simulink model "test_yL_epsL"  (R2018a)
settings: Solver=ode23  StartTime=0.0  StopTime=tend  FixedStep=0.01  RelTol=1e-3  EnableMultiTasking=on
values from neighbouring files (symbols this model uses):
  delta = @(u) 0.0015*(u-t0)*(u>t0) - 0.0035*(u-t1)*(u>t1)    [test_yL_epsL_.m]
undefined symbols (not defined in the file or in its folder): pin
libraries: SLlib_lka_thesis x6, simulink_extras x1, simulink x1
settings Model: Creator=Georg  LastModifiedBy=georgnestlinger
settings DataIOCC: LimitDataPoints=on  SaveFormat=Array  SignalLoggingSaveFormat=ModelDataLogs
settings OptimizationCC: DefaultParameterBehavior=Inlined  ExpressionDepthLimit=2147483647  LifeSpan=inf
settings DebuggingCC: UnderspecifiedInitializationDetection=Classic  MergeDetectMultiDrivingBlocksExec=none  StateNameClashWarn=warning  SFUnexpectedBacktrackingDiag=warning  SFNoUnconditionalDefaultTransitionDiag=warning  SFExecutionAtInitializationDiag=none
settings HardwareCC: ProdBitPerPointer=32  ProdBitPerSizeT=32  ProdBitPerPtrDiffT=32  ProdLargestAtomicFloat=None  ProdIntDivRoundTo=Undefined  ProdEndianess=Unspecified  ProdWordSize=32  ProdHWDeviceType=32-bit Generic
settings ModelReferenceCC: PropagateSignalLabelsOutOfModel=off
settings CodeAppCC: StateflowObjectComments=on
settings GRTTargetCC: TargetLangStandard=C89/C90 (ANSI)  GeneratePreprocessorConditionals=Disable all  CombineOutputUpdateFcns=off  GRTInterface=on
settings ConfigComp: CovMetricSettings=dw  CovHtmlReporting=on  CovSaveCumulativeToWorkspaceVar=on  CovSaveSingleToWorkspaceVar=on  CovExternalEMLEnable=off

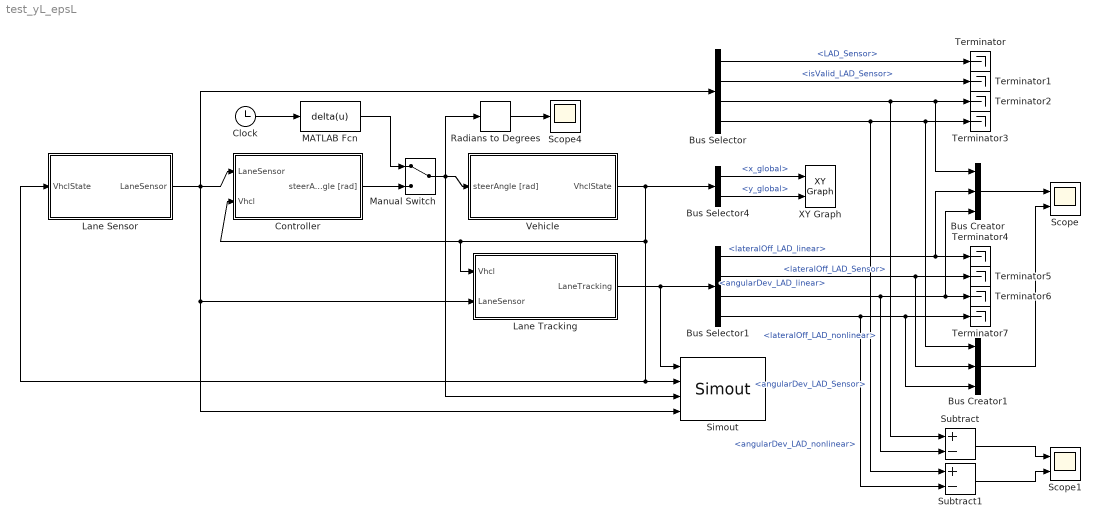
== system test_yL_epsL ==
  Bus Creator : BusCreator  Inputs=3
  Bus Creator1 : BusCreator  Inputs=3
  Bus Selector : BusSelector  OutputSignals=LAD_Sensor,isValid_LAD_Sensor,lateralOff_LAD_Sensor,angularDev_LAD_Sensor
  Bus Selector1 : BusSelector  OutputSignals=lateralOff_LAD_linear,angularDev_LAD_linear,lateralOff_LAD_nonlinear,angularDev_LAD_nonlinear
  Bus Selector4 : BusSelector  OutputSignals=x_global,y_global
  Clock : Clock
  Controller : Subsystem
  Lane Sensor : Subsystem
  Lane Tracking : Subsystem
  MATLAB Fcn : MATLABFcn  MATLABFcn=delta(u)
  Manual Switch : ManualSwitch
  Radians to Degrees : simulink_extras/Transformations/Radians to Degrees
  Scope : Scope  NumInputPorts=2
  Scope1 : Scope  NumInputPorts=2
  Scope4 : Scope
  Simout : SLlib_lka_thesis/Misc/Simout
  Subtract : Sum  Inputs=+-
  Subtract1 : Sum  Inputs=+-
  Terminator{,1..7} (8 alike) : Terminator
  Vehicle : Subsystem
  XY Graph : simulink/Sinks/XY Graph  xmin=-50  xmax=700  ymin=-10  ymax=600  st=-1
  wires:
  MATLAB Fcn/1 -> Manual Switch/1
  Clock/1 -> MATLAB Fcn/1
  Radians to Degrees/1 -> Scope4/1
  Manual Switch/1 -> Vehicle/1(steerAngle [rad]), Radians to Degrees/1, Simout/3
  Controller/1(steerAngle [rad]) -> Manual Switch/2
  Vehicle/1(VhclState) -> Bus Selector4/1, Lane Tracking/1(Vhcl), Controller/2(Vhcl), Simout/2, Lane Sensor/1(VhclState)
  Lane Sensor/1(LaneSensor) -> Controller/1(LaneSensor), Bus Selector/1, Lane Tracking/2(LaneSensor), Simout/4
  Bus Selector4/1 -> XY Graph/1  "<x_global>"
  Bus Selector4/2 -> XY Graph/2  "<y_global>"
  Bus Creator1/1 -> Scope/2
  Bus Creator/1 -> Scope/1
  Lane Tracking/1(LaneTracking) -> Bus Selector1/1, Simout/1
  Bus Selector/1 -> Terminator/1  "<LAD_Sensor>"
  Bus Selector/2 -> Terminator1/1  "<isValid_LAD_Sensor>"
  Bus Selector/3 -> Terminator2/1, Bus Creator/1, Subtract/1  "<lateralOff_LAD_Sensor>"
  Bus Selector/4 -> Terminator3/1, Bus Creator1/1, Subtract1/1  "<angularDev_LAD_Sensor>"
  Bus Selector1/1 -> Terminator4/1, Bus Creator/2  "<lateralOff_LAD_linear>"
  Bus Selector1/2 -> Terminator5/1, Bus Creator1/2  "<angularDev_LAD_linear>"
  Bus Selector1/3 -> Terminator6/1, Bus Creator/3, Subtract/2  "<lateralOff_LAD_nonlinear>"
  Bus Selector1/4 -> Terminator7/1, Bus Creator1/3, Subtract1/2  "<angularDev_LAD_nonlinear>"
  Subtract1/1 -> Scope1/2
  Subtract/1 -> Scope1/1

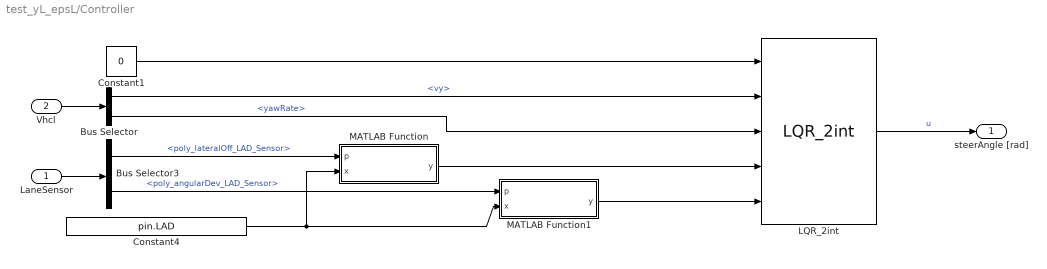
== system test_yL_epsL/Controller ==
  LaneSensor : Inport
  Vhcl : Inport  Port=2
  Bus Selector : BusSelector  OutputSignals=vy,yawRate
  Bus Selector3 : BusSelector  OutputSignals=poly_lateralOff_LAD_Sensor,poly_angularDev_LAD_Sensor
  Constant1 : Constant  Value=0
  Constant4 : Constant  Value=pin.LAD
  LQR_2int : SLlib_lka_thesis/LKA-Controller/LQR_2int
  MATLAB Function : MATLAB Function  TreatAsAtomicUnit=on
  MATLAB Function1 : MATLAB Function  TreatAsAtomicUnit=on
  steerAngle [rad] : Outport
  wires:
  Constant1/1 -> LQR_2int/1
  MATLAB Function/1(y) -> LQR_2int/4
  MATLAB Function1/1(y) -> LQR_2int/5
  Constant4/1 -> MATLAB Function1/2(x), MATLAB Function/2(x)
  LaneSensor/1 -> Bus Selector3/1
  LQR_2int/1 -> steerAngle [rad]/1  "u"
  Bus Selector3/1 -> MATLAB Function/1(p)  "<poly_lateralOff_LAD_Sensor>"
  Bus Selector3/2 -> MATLAB Function1/1(p)  "<poly_angularDev_LAD_Sensor>"
  Vhcl/1 -> Bus Selector/1
  Bus Selector/1 -> LQR_2int/2  "<vy>"
  Bus Selector/2 -> LQR_2int/3  "<yawRate>"

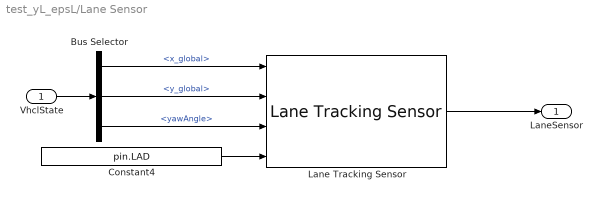
== system test_yL_epsL/Lane Sensor ==
  VhclState : Inport
  Bus Selector : BusSelector  OutputSignals=x_global,y_global,yawAngle
  Constant4 : Constant  Value=pin.LAD
  Lane Tracking Sensor : SLlib_lka_thesis/Lane Tracking/Lane Tracking Sensor
  LaneSensor : Outport
  wires:
  Lane Tracking Sensor/1 -> LaneSensor/1
  VhclState/1 -> Bus Selector/1
  Bus Selector/1 -> Lane Tracking Sensor/1  "<x_global>"
  Bus Selector/2 -> Lane Tracking Sensor/2  "<y_global>"
  Bus Selector/3 -> Lane Tracking Sensor/3  "<yawAngle>"
  Constant4/1 -> Lane Tracking Sensor/4

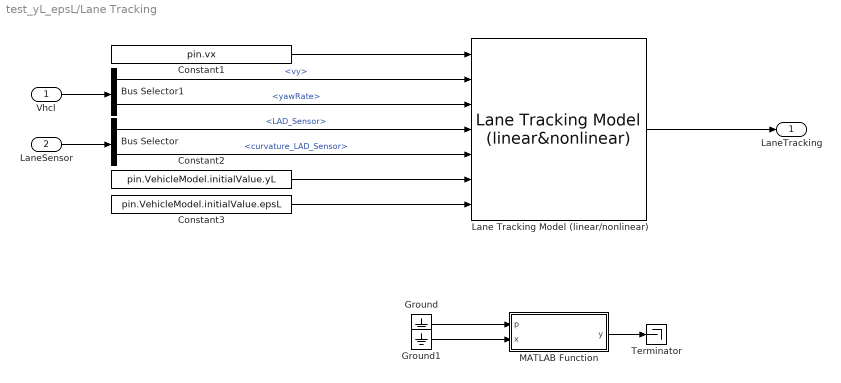
== system test_yL_epsL/Lane Tracking ==
  Vhcl : Inport
  LaneSensor : Inport  Port=2
  Bus Selector : BusSelector  OutputSignals=LAD_Sensor,curvature_LAD_Sensor
  Bus Selector1 : BusSelector  OutputSignals=vy,yawRate
  Constant1 : Constant  Value=pin.vx
  Constant2 : Constant  Value=pin.VehicleModel.initialValue.yL
  Constant3 : Constant  Value=pin.VehicleModel.initialValue.epsL
  Ground : Ground
  Ground1 : Ground
  Lane Tracking Model (linear/nonlinear) : SLlib_lka_thesis/Lane Tracking/Lane Tracking Model (linear&nonlinear)
  MATLAB Function : MATLAB Function  TreatAsAtomicUnit=on
  Terminator : Terminator
  LaneTracking : Outport
  wires:
  LaneSensor/1 -> Bus Selector/1
  Constant2/1 -> Lane Tracking Model (linear/nonlinear)/6
  Constant3/1 -> Lane Tracking Model (linear/nonlinear)/7
  Vhcl/1 -> Bus Selector1/1
  Constant1/1 -> Lane Tracking Model (linear/nonlinear)/1
  Bus Selector1/1 -> Lane Tracking Model (linear/nonlinear)/2  "<vy>"
  Bus Selector1/2 -> Lane Tracking Model (linear/nonlinear)/3  "<yawRate>"
  Bus Selector/1 -> Lane Tracking Model (linear/nonlinear)/4  "<LAD_Sensor>"
  Bus Selector/2 -> Lane Tracking Model (linear/nonlinear)/5  "<curvature_LAD_Sensor>"
  Lane Tracking Model (linear/nonlinear)/1 -> LaneTracking/1
  Ground/1 -> MATLAB Function/1(p)
  Ground1/1 -> MATLAB Function/2(x)
  MATLAB Function/1(y) -> Terminator/1

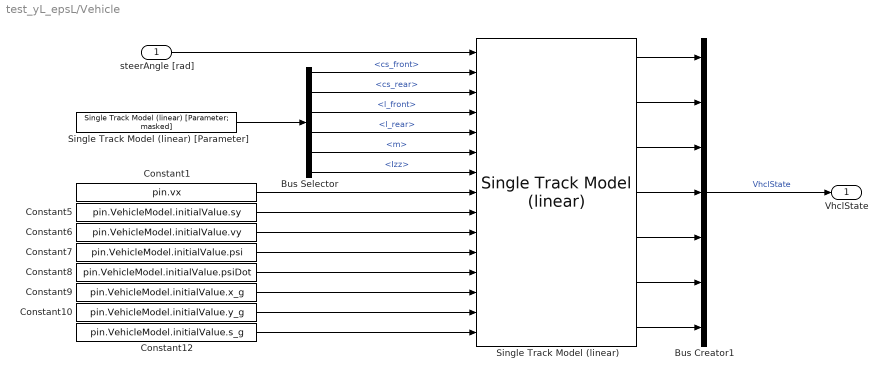
== system test_yL_epsL/Vehicle ==
  steerAngle [rad] : Inport
  Bus Creator1 : BusCreator  Inputs=7
  Bus Selector : BusSelector  OutputSignals=cs_front,cs_rear,l_front,l_rear,m,Izz
  Constant1 : Constant  Value=pin.vx
  Constant10 : Constant  Value=pin.VehicleModel.initialValue.y_g
  Constant12 : Constant  Value=pin.VehicleModel.initialValue.s_g
  Constant5 : Constant  Value=pin.VehicleModel.initialValue.sy
  Constant6 : Constant  Value=pin.VehicleModel.initialValue.vy
  Constant7 : Constant  Value=pin.VehicleModel.initialValue.psi
  Constant8 : Constant  Value=pin.VehicleModel.initialValue.psiDot
  Constant9 : Constant  Value=pin.VehicleModel.initialValue.x_g
  Single Track Model (linear) : SLlib_lka_thesis/Vehicle Models/Single Track Models/Single Track Model (linear)
  Single Track Model (linear) [Parameter] : SLlib_lka_thesis/Vehicle Models ext./Single Track Model (linear) [Parameter; masked]  cs_front=pin.VehicleModel.parameter.cs_front  cs_rear=pin.VehicleModel.parameter.cs_rear  l_front=pin.VehicleModel.parameter.l_front  l_rear=pin.VehicleModel.parameter.l_rear  m=pin.VehicleModel.parameter.m  Izz=pin.VehicleModel.parameter.Izz
  VhclState : Outport
  wires:
  Constant1/1 -> Single Track Model (linear)/8
  steerAngle [rad]/1 -> Single Track Model (linear)/1
  Single Track Model (linear) [Parameter]/1 -> Bus Selector/1
  Constant5/1 -> Single Track Model (linear)/9
  Constant6/1 -> Single Track Model (linear)/10
  Constant7/1 -> Single Track Model (linear)/11
  Constant8/1 -> Single Track Model (linear)/12
  Constant9/1 -> Single Track Model (linear)/13
  Constant10/1 -> Single Track Model (linear)/14
  Constant12/1 -> Single Track Model (linear)/15
  Bus Creator1/1 -> VhclState/1  "VhclState"
  Single Track Model (linear)/1 -> Bus Creator1/1
  Single Track Model (linear)/2 -> Bus Creator1/2
  Single Track Model (linear)/3 -> Bus Creator1/3
  Single Track Model (linear)/4 -> Bus Creator1/4
  Single Track Model (linear)/5 -> Bus Creator1/5
  Single Track Model (linear)/6 -> Bus Creator1/6
  Single Track Model (linear)/7 -> Bus Creator1/7
  Bus Selector/1 -> Single Track Model (linear)/2  "<cs_front>"
  Bus Selector/2 -> Single Track Model (linear)/3  "<cs_rear>"
  Bus Selector/3 -> Single Track Model (linear)/4  "<l_front>"
  Bus Selector/4 -> Single Track Model (linear)/5  "<l_rear>"
  Bus Selector/5 -> Single Track Model (linear)/6  "<m>"
  Bus Selector/6 -> Single Track Model (linear)/7  "<Izz>"

== matlab function test_yL_epsL/Controller/MATLAB Function ==
  data: p input; y output; x input
function y = polyVal(p,x)
%#codegen

y = polyval(p,x);

== matlab function test_yL_epsL/Controller/MATLAB Function1 ==
  data: p input; y output; x input
function y = polyVal(p,x)
%#codegen

y = polyval(p,x);

== matlab function test_yL_epsL/Lane Tracking/MATLAB Function ==
  data: p input; y output; x input
function y = polyVal(p,x)
%#codegen

y = polyval(p,x);
